simulink model "FM_Modulation"  (R2019a)
settings: Solver=VariableStepAuto  StartTime=0.0  StopTime=5  RelTol=1e-3
libraries: commanapbnd3 x2, dsparch4 x1
settings Model: Creator=Dawson  LastModifiedBy=Dawson

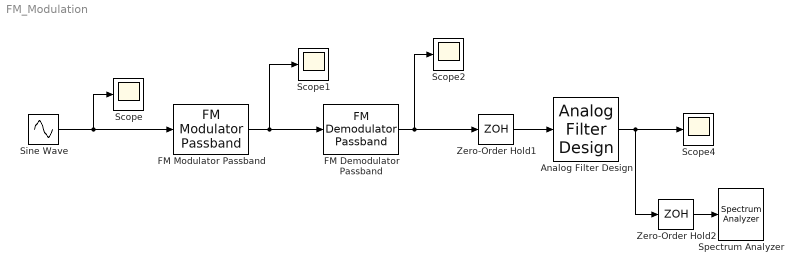
== system FM_Modulation ==
  Analog Filter Design : dsparch4/Analog Filter Design  method=Butterworth  filttype=Lowpass  N=8  Wlo=30  Whi=80  Rp=2  Rs=40
  FM Demodulator Passband : commanapbnd3/FM Demodulator Passband  Fc=5000  Ph=0  Kc=50  Ho=100
      settings: SourceProductName=Communications Toolbox  SourceProductBaseCode=CM
  FM Modulator Passband : commanapbnd3/FM Modulator Passband  Fc=50000  Ph=0  Kc=50
      settings: SourceProductName=Communications Toolbox  SourceProductBaseCode=CM
  Scope{,1..2,4} (4 alike) : Scope
  Sine Wave : Sin  Frequency=1000  SampleTime=1/5000
  Spectrum Analyzer : SpectrumAnalyzer
  Zero-Order Hold1 : ZeroOrderHold  SampleTime=1/5000
  Zero-Order Hold2 : ZeroOrderHold  SampleTime=1/5000
  wires:
  Sine Wave/1 -> Scope/1, FM Modulator Passband/1
  FM Modulator Passband/1 -> FM Demodulator Passband/1, Scope1/1
  FM Demodulator Passband/1 -> Zero-Order Hold1/1, Scope2/1
  Zero-Order Hold1/1 -> Analog Filter Design/1
  Analog Filter Design/1 -> Zero-Order Hold2/1, Scope4/1
  Zero-Order Hold2/1 -> Spectrum Analyzer/1
